simulink model "StateSpace_DifferenceEq"  (R2023b)
settings: Solver=FixedStepDiscrete  StartTime=T_start  StopTime=T_stop  FixedStep=Ts  RelTol=1e-3
undefined symbols (not defined in the file): u_Om1, u_Om2, u_Om3, x1_0, x2_0, x3_0
settings Model: Creator=fenu  LastModifiedBy=alberto
settings DataIOCC: SaveFormat=Array  SaveState=on  SignalLogging=off  DSMLogging=off
settings OptimizationCC: ReuseModelBlockBuffer=off

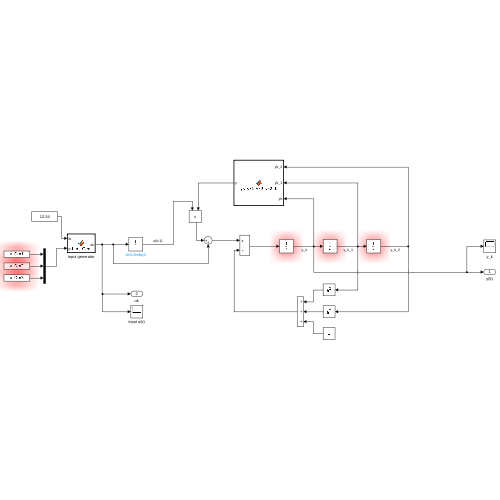
[thumbnail: Simulink's stored preview of the top-level diagram]
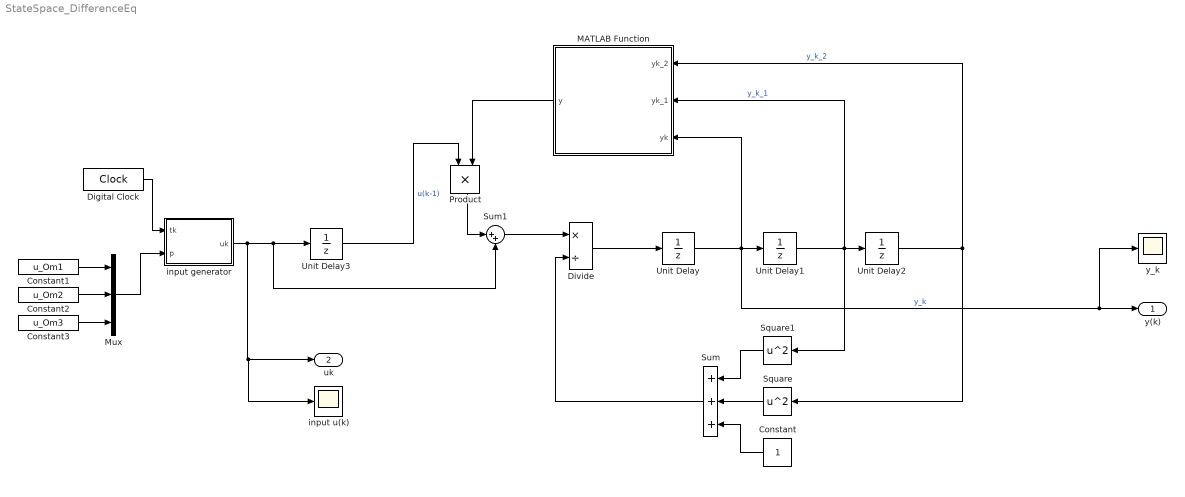
== system StateSpace_DifferenceEq ==
  Constant : Constant
  Constant1 : Constant  Value=u_Om1  SampleTime=1
  Constant2 : Constant  Value=u_Om2  SampleTime=1
  Constant3 : Constant  Value=u_Om3  SampleTime=1
  Digital Clock : DigitalClock
  Divide : Product  Inputs=*/
  MATLAB Function : MATLAB Function  TreatAsAtomicUnit=on
  Mux : Mux  Inputs=3
  Product : Product
  Square : Math  Operator=square
  Square1 : Math  Operator=square
  Sum : Sum  Inputs=+++
  Sum1 : Sum  Inputs=|++
  Unit Delay : UnitDelay  InitialCondition=x3_0  SampleTime=-1  HasFrameUpgradeWarning=on
  Unit Delay1 : UnitDelay  InitialCondition=x2_0  SampleTime=-1  HasFrameUpgradeWarning=on
  Unit Delay2 : UnitDelay  InitialCondition=x1_0  SampleTime=-1  HasFrameUpgradeWarning=on
  Unit Delay3 : UnitDelay  SampleTime=-1  HasFrameUpgradeWarning=on
  input generator : MATLAB Function  TreatAsAtomicUnit=on
  input u(k) : Scope
  y_k : Scope
  y(k) : Outport
  uk : Outport  Port=2
  wires:
  Unit Delay/1 -> MATLAB Function/3(yk), y_k/1, y(k)/1, Unit Delay1/1  "y_k"
  Unit Delay2/1 -> MATLAB Function/1(yk_2), Square/1  "y_k_2"
  Unit Delay1/1 -> MATLAB Function/2(yk_1), Unit Delay2/1, Square1/1  "y_k_1"
  Square/1 -> Sum/2
  Square1/1 -> Sum/1
  Constant/1 -> Sum/3
  MATLAB Function/1(y) -> Product/2
  Unit Delay3/1 -> Product/1  "u(k-1)"
  Product/1 -> Sum1/1
  input generator/1(uk) -> input u(k)/1, uk/1, Sum1/2, Unit Delay3/1
  Divide/1 -> Unit Delay/1
  Sum1/1 -> Divide/1
  Sum/1 -> Divide/2
  Digital Clock/1 -> input generator/1(tk)
  Mux/1 -> input generator/2(p)
  Constant1/1 -> Mux/1
  Constant2/1 -> Mux/2
  Constant3/1 -> Mux/3

== matlab function StateSpace_DifferenceEq/MATLAB Function ==
  data: yk_2 input; yk_1 input; yk input; y output
function y = yk_yk1_yk2_yk2_1(yk_2, yk_1, yk)

y = yk*yk_1*yk_2*(yk_2-1);

== matlab function StateSpace_DifferenceEq/input generator ==
  data: tk input; uk output; p input
function uk = InputGen(tk, p)
Om1 = p(1);
Om2 = p(2);
Om3 = p(3);

uk = sin(Om1*tk)+sin(Om2*tk)-cos(Om3*tk);
